simulink model "val_plant"  (R2026a)
settings: Solver=VariableStepAuto  StopTime=100
libraries: lib_plant x1
settings Model: Creator=alessandro-nardin  LastModifiedBy=alessandro-nardin

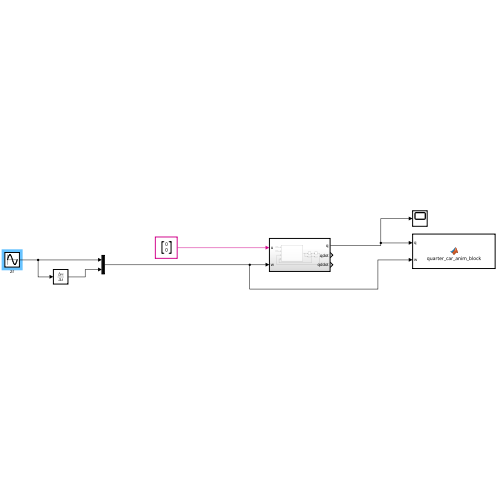
[thumbnail: Simulink's stored preview of the top-level diagram]
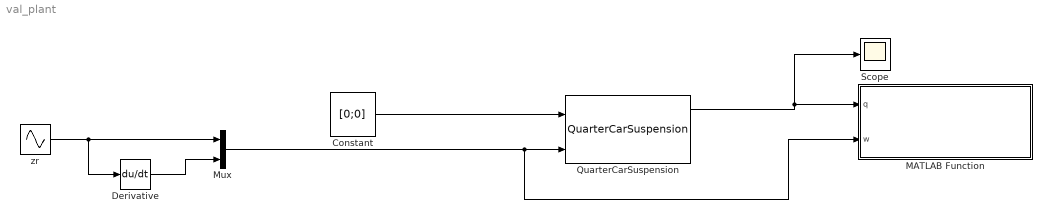
== system val_plant ==
  Constant : Constant  Value=[0;0]  VectorParams1D=off
  Derivative : Derivative
  MATLAB Function : MATLAB Function  TreatAsAtomicUnit=on
  Mux : Mux  Inputs=2
  QuarterCarSuspension : lib_plant/QuarterCarSuspension  SystemSampleTime=-1  VariantActivationTime=update diagram  EmptyChoice=off  PassThrough=off  PassThroughVariantControl=(default)  EmptyChoiceVariantControl=(default)  AllowFlexibleInterface=on  Latency=0  AutoFrameSizeCalculation=off
      settings: SourceProductName=Lib Plant
  Scope : Scope
      settings: ActiveDisplayYMinimum=-0.25608885933474745  ActiveDisplayYMaximum=0.098043047230608721
  zr : Sin  Amplitude=2  Frequency=9  SampleTime=0
  wires:
  Constant/1 -> QuarterCarSuspension/1
  Mux/1 -> MATLAB Function/2(w), QuarterCarSuspension/2
  QuarterCarSuspension/1 -> Scope/1, MATLAB Function/1(q)
  Derivative/1 -> Mux/2
  zr/1 -> Derivative/1, Mux/1

== matlab function val_plant/MATLAB Function ==
  data: q input; w input
function quarter_car_anim_block(q,w)
%#codegen

coder.extrinsic('figure','axes','hold','grid','box','xlim','ylim', ...
                'ylabel','title','line','plot','text','set','drawnow');

persistent isInit
persistent fig ax
persistent hCar hWheel hRoad
persistent hLine1 hLine2
persistent hTextCar hTextWheel hTextRoad

% ---------------------------
% USER SETTINGS
% ---------------------------
zr0 = 0.0;      % road equilibrium height [cm]
zu0 = 50;      % wheel equilibrium height [cm]
zs0 = 100;      % car equilibrium height [cm]

yMargin = 1.0;  % visible vertical margin [cm]

xCenter = 0.0;  % common x position
xText   = 0.08; % label offset
xSpan   = 0.35; % x axis half-width

markerSize = 14;

roadColor  = [0.20 0.20 0.20];
wheelColor = [0.47 0.67 0.19];
carColor   = [0.85 0.33 0.10];

lineColor1 = [0.49 0.18 0.56]; % road-wheel
lineColor2 = [0.00 0.45 0.74]; % wheel-car

% extract inputs
zs = q(1);
zu = q(2);
zr = w(1);

% Current positions
yRoad  = zr0 + zr;
yWheel = zu0 + zu;
yCar   = zs0 + zs;

% First call: create everything
if isempty(isInit)
    fig = figure('Name','Quarter Car Animation', ...
                 'NumberTitle','off', ...
                 'Color','w');

    ax = axes('Parent', fig);
    hold(ax,'on');
    grid(ax,'on');
    box(ax,'on');

    xlim(ax,[-xSpan xSpan]);
    ylim(ax,[min([zr0 zu0 zs0]) - yMargin, max([zr0 zu0 zs0]) + yMargin]);
    ylabel(ax,'Vertical position [m]');
    title(ax,'Quarter Car Suspension Animation');

    hLine1 = line(ax, [xCenter xCenter], [yRoad yWheel], ...
        'Color', lineColor1, 'LineWidth', 3);

    hLine2 = line(ax, [xCenter xCenter], [yWheel yCar], ...
        'Color', lineColor2, 'LineWidth', 3);

    hRoad = plot(ax, xCenter, yRoad, 'o', ...
        'MarkerSize', markerSize, ...
        'MarkerFaceColor', roadColor, ...
        'MarkerEdgeColor', 'k');

    hWheel = plot(ax, xCenter, yWheel, 'o', ...
        'MarkerSize', markerSize, ...
        'MarkerFaceColor', wheelColor, ...
        'MarkerEdgeColor', 'k');

    hCar = plot(ax, xCenter, yCar, 'o', ...
        'MarkerSize', markerSize, ...
        'MarkerFaceColor', carColor, ...
        'MarkerEdgeColor', 'k');

    hTextRoad = text(ax, xCenter + xText, yRoad, 'zr', ...
        'VerticalAlignment','middle', 'FontSize', 11);

    hTextWheel = text(ax, xCenter + xText, yWheel, 'zu', ...
        'VerticalAlignment','middle', 'FontSize', 11);

    hTextCar = text(ax, xCenter + xText, yCar, 'zs', ...
        'VerticalAlignment','middle', 'FontSize', 11);

    isInit = true;
    drawnow;
else
    set(hLine1, 'XData', [xCenter xCenter], 'YData', [yRoad yWheel]);
    set(hLine2, 'XData', [xCenter xCenter], 'YData', [yWheel yCar]);

    set(hRoad,  'XData', xCenter, 'YData', yRoad);
    set(hWheel, 'XData', xCenter, 'YData', yWheel);
    set(hCar,   'XData', xCenter, 'YData', yCar);

    set(hTextRoad,  'Position', [xCenter + xText, yRoad, 0]);
    set(hTextWheel, 'Position', [xCenter + xText, yWheel, 0]);
    set(hTextCar,   'Position', [xCenter + xText, yCar, 0]);

    drawnow limitrate;
end
